simulink model "Bi_uni"  (R2017a)
settings: Solver=ode23s  StartTime=0.0  StopTime=0.5  MaxStep=1e-6  RelTol=1e-3  EnableMultiTasking=on
libraries: powerlib x19, powerlib_meascontrol x5
settings Model: Creator=Amr  LastModifiedBy=lenovo 520
settings DataIOCC: LimitDataPoints=on  SaveFormat=Array
settings OptimizationCC: LifeSpan=inf
settings DebuggingCC: SFUnexpectedBacktrackingDiag=warning  SFNoUnconditionalDefaultTransitionDiag=warning  SFExecutionAtInitializationDiag=none
settings HardwareCC: ProdBitPerPointer=32  ProdBitPerSizeT=32  ProdBitPerPtrDiffT=32  ProdLargestAtomicFloat=None  ProdIntDivRoundTo=Undefined  ProdEndianess=Unspecified  ProdWordSize=32  ProdHWDeviceType=32-bit Generic
settings ModelReferenceCC: PropagateSignalLabelsOutOfModel=off
settings GRTTargetCC: TargetLangStandard=C89/C90 (ANSI)  GeneratePreprocessorConditionals=Disable all
settings ConfigComp: CovMetricSettings=dw  CovHtmlReporting=on  CovSaveCumulativeToWorkspaceVar=on  CovSaveSingleToWorkspaceVar=on  CovExternalEMLEnable=off

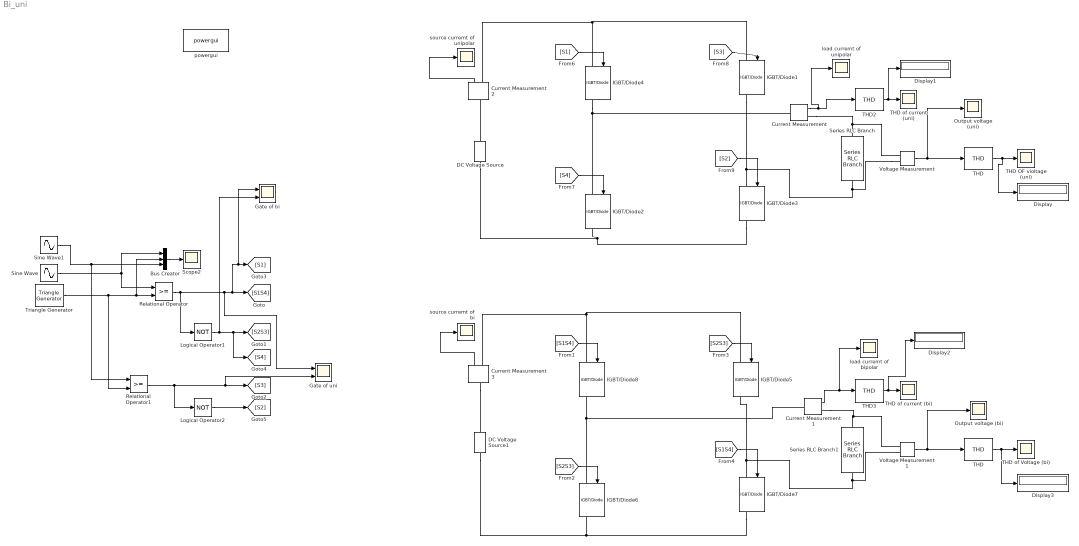
== system Bi_uni ==
  Bus Creator : BusCreator  Inputs=3
  Current Measurement{,1..3} (4 alike) : powerlib/Measurements/Current Measurement  PhasorSimulation=off  OutputType=Complex  PSBequivalent=0
  DC Voltage Source : powerlib/Electrical Sources/DC Voltage Source  Amplitude=200  Measurements=None
  DC Voltage Source1 : powerlib/Electrical Sources/DC Voltage Source  Amplitude=200  Measurements=None
  Display{,1..3} (4 alike) : Display
  Gate of bi : Scope  NumInputPorts=2
  Gate of uni : Scope  NumInputPorts=2
  IGBT/Diode{1..8} (8 alike) : powerlib/Power Electronics/IGBT//Diode  Ron=1e-3  Rs=1e5  Cs=inf  Measurements=on
  Logical Operator1 : Logic  Operator=NOT  Inputs=1  AllPortsSameDT=off  OutDataTypeStr=boolean
  Logical Operator2 : Logic  Operator=NOT  Inputs=1  AllPortsSameDT=off  OutDataTypeStr=boolean
  "Output voltage (bi) " : Scope
  "Output voltage (uni) " : Scope
  Relational Operator : RelationalOperator  OutDataTypeStr=boolean  RndMeth=Nearest
  Relational Operator1 : RelationalOperator  OutDataTypeStr=boolean  RndMeth=Nearest
  Scope2 : Scope
  Series RLC Branch : powerlib/Elements/Series RLC Branch  LConnTagsString=__new0  RConnTagsString=__new0  BranchType=RL  Resistance=1  Inductance=1e-3  SetiL0=off  InitialCurrent=0  Capacitance=1e-6  Setx0=off  InitialVoltage=0  Measurements=None
  Series RLC Branch1 : powerlib/Elements/Series RLC Branch  LConnTagsString=__new0  RConnTagsString=__new0  BranchType=RL  Resistance=1  Inductance=1e-3  SetiL0=off  InitialCurrent=0  Capacitance=1e-6  Setx0=off  InitialVoltage=0  Measurements=None
  Sine Wave : Sin  Frequency=50*2*pi  SampleTime=0
  Sine Wave1 : Sin  Frequency=50*2*pi  Phase=pi  SampleTime=0
  THD : powerlib_meascontrol/Measurements/THD  Freq=50  Ts=0
  "THD " : powerlib_meascontrol/Measurements/THD  Freq=50  Ts=0
  "THD OF violtage (uni) " : Scope
  "THD of Voltage (bi) " : Scope
  "THD of current (bi) " : Scope
  "THD of current (uni) " : Scope
  THD2 : powerlib_meascontrol/Measurements/THD  Freq=50  Ts=0
  THD3 : powerlib_meascontrol/Measurements/THD  Freq=50  Ts=0
  Triangle Generator : powerlib_meascontrol/Pulse & Signal Generators/Triangle Generator  Freq=50*21  Phase=0  Ts=0
  Voltage Measurement : powerlib/Measurements/Voltage Measurement  PhasorSimulation=off  OutputType=Complex  PSBequivalent=0
  Voltage Measurement1 : powerlib/Measurements/Voltage Measurement  PhasorSimulation=off  OutputType=Complex  PSBequivalent=0
  "load curremt of bipolar " : Scope
  load curremt of unipolar : Scope
  powergui : powerlib/powergui  Priority=1  SimulationMode=Continuous  SampleTime=50e-6  frequency=60  Iterations=50  frequencyindice=0  Pbase=100e6  ErrMax=1e-4  UnitsV=kV  UnitsW=MW  buscounter=0  FunctionMessages=off  echomessages=off  EnableUseOfTLC=off  CurrentSourceSwitches=off  DisableSnubberDevices=off  DisableRonSwitches=off  DisableVfSwitches=off  DisplayEquations=off  SolverType=Tustin/Backward Euler (TBE)  Interpol=off  ExternalGateDelay=off  methode=off  Ts=100  x0status=blocks  SPID=off  SwTol=0  HookPort=off  RestoreLinks=warning  ResistiveCurrentMeasurement=off  Frange=[0:2:500]  Ylog=off  Xlog=on  ShowGrid=off  save=off  variable=ZData  structure=ScopeData2  ZoomFFT=off  StartTime=0.02  cycles=10  DisplayStyle=1  fundamental=50  FreqAxis=on  MaxFrequency=10000  frequencyindicesteady=1  RmsSteady=1  display=off
  source curremt of bi : Scope
  source curremt of unipolar : Scope
  wires:
  Sine Wave/1 -> Bus Creator/1, Relational Operator/1
  Triangle Generator/1 -> Relational Operator1/2, Bus Creator/2, Relational Operator/2
  Relational Operator/1 -> Gate of uni/1, Gate of bi/1, [S1], [S1S4], Logical Operator1/1
  Logical Operator1/1 -> Gate of bi/2, [S4], [S2S3]
  [S1] -> IGBT/Diode4/1
  [S3] -> IGBT/Diode1/1
  [S4] -> IGBT/Diode2/1
  [S2] -> IGBT/Diode3/1
  Voltage Measurement/1 -> "Output voltage (uni) "/1, THD/1
  THD/1 -> Display/1, "THD OF violtage (uni) "/1
  [S1S4] -> IGBT/Diode7/1
  Voltage Measurement1/1 -> "Output voltage (bi) "/1, "THD "/1
  [S1S4] -> IGBT/Diode8/1
  [S2S3] -> IGBT/Diode6/1
  [S2S3] -> IGBT/Diode5/1
  "THD "/1 -> Display3/1, "THD of Voltage (bi) "/1
  Bus Creator/1 -> Scope2/1
  Sine Wave1/1 -> Bus Creator/3, Relational Operator1/1
  Relational Operator1/1 -> Gate of uni/2, [S3], Logical Operator2/1
  Logical Operator2/1 -> [S2]
  Current Measurement/1 -> load curremt of unipolar/1, THD2/1
  Current Measurement1/1 -> "load curremt of bipolar "/1, THD3/1
  THD3/1 -> Display2/1, "THD of current (bi) "/1
  Current Measurement2/1 -> source curremt of unipolar/1
  Current Measurement3/1 -> source curremt of bi/1
  THD2/1 -> Display1/1, "THD of current (uni) "/1
  connections:
  IGBT/Diode4/RConn1 -- IGBT/Diode2/LConn1 -- Current Measurement/LConn1
  Voltage Measurement/LConn2 -- Series RLC Branch/RConn1 -- IGBT/Diode1/RConn1 -- IGBT/Diode3/LConn1
  IGBT/Diode4/LConn1 -- Current Measurement2/RConn1 -- IGBT/Diode1/LConn1
  IGBT/Diode2/RConn1 -- DC Voltage Source/LConn1 -- IGBT/Diode3/RConn1
  IGBT/Diode7/RConn1 -- DC Voltage Source1/LConn1 -- IGBT/Diode6/RConn1
  IGBT/Diode6/LConn1 -- Current Measurement1/LConn1 -- IGBT/Diode8/RConn1
  IGBT/Diode7/LConn1 -- Voltage Measurement1/LConn2 -- Series RLC Branch1/RConn1 -- IGBT/Diode5/RConn1
  IGBT/Diode8/LConn1 -- Current Measurement3/RConn1 -- IGBT/Diode5/LConn1
  Series RLC Branch/LConn1 -- Current Measurement/RConn1 -- Voltage Measurement/LConn1
  Series RLC Branch1/LConn1 -- Current Measurement1/RConn1 -- Voltage Measurement1/LConn1
  DC Voltage Source/RConn1 -- Current Measurement2/LConn1
  Current Measurement3/LConn1 -- DC Voltage Source1/RConn1
